simulink model "SimuContinu"  (Simulink 8.3)
settings: Solver=ode45  StartTime=0.0  StopTime=10.0  RelTol=1e-3
libraries: cstblocks x2, simulink x1
settings Model: Creator=cadenat  LastModifiedBy=2asri13
settings OptimizationCC: ExpressionDepthLimit=2147483647
settings DebuggingCC: FcnCallInpInsideContextMsg=UseLocalSettings

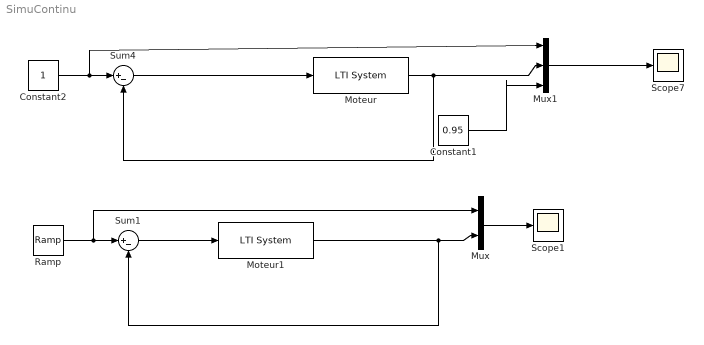
== system SimuContinu ==
  Constant1 : Constant  Value=0.95
  Constant2 : Constant
  Moteur : cstblocks/LTI System  sys=G  IC=[]
  Moteur1 : cstblocks/LTI System  sys=G  IC=[]
  Mux : Mux  Inputs=2
  Mux1 : Mux  Inputs=3
  Ramp : simulink/Sources/Ramp  slope=1  start=0  X0=0
  Scope1 : Scope
  Scope7 : Scope
  Sum1 : Sum  Inputs=|+-  SaturateOnIntegerOverflow=on  InputSameDT=on  OutDataTypeStr=Inherit: Same as first input
  Sum4 : Sum  Inputs=|+-  SaturateOnIntegerOverflow=on  InputSameDT=on  OutDataTypeStr=Inherit: Same as first input
  wires:
  Sum4/1 -> Moteur/1
  Moteur/1 -> Mux1/2, Sum4/2
  Constant2/1 -> Mux1/1, Sum4/1
  Sum1/1 -> Moteur1/1
  Moteur1/1 -> Sum1/2, Mux/2
  Ramp/1 -> Sum1/1, Mux/1
  Mux/1 -> Scope1/1
  Mux1/1 -> Scope7/1
  Constant1/1 -> Mux1/3
